simulink library "Blokk_Konyvtar"  (R2024b)
settings: Solver=VariableStepAuto  StartTime=0.0  StopTime=10.0  RelTol=1e-3
undefined symbols (not defined in the file or in its folder): __PRM__SERIALIZED__DATA__, Encoder, Sebessegmero
libraries: stm32f4xxblockslib x16, simulink x13, stm32blockslib x3, simulink_extras x2
settings Model: Creator=Asus  LastModifiedBy=Asus

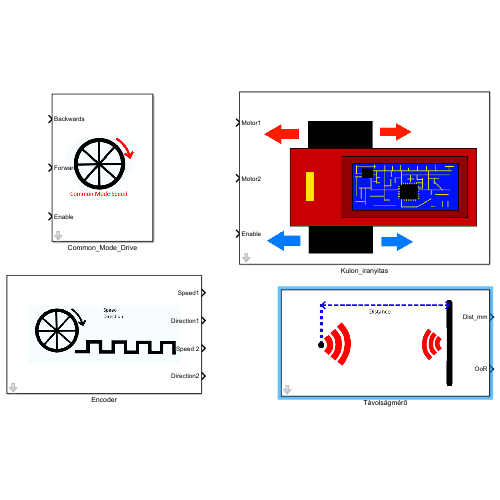
[thumbnail: Simulink's stored preview of the top-level diagram]
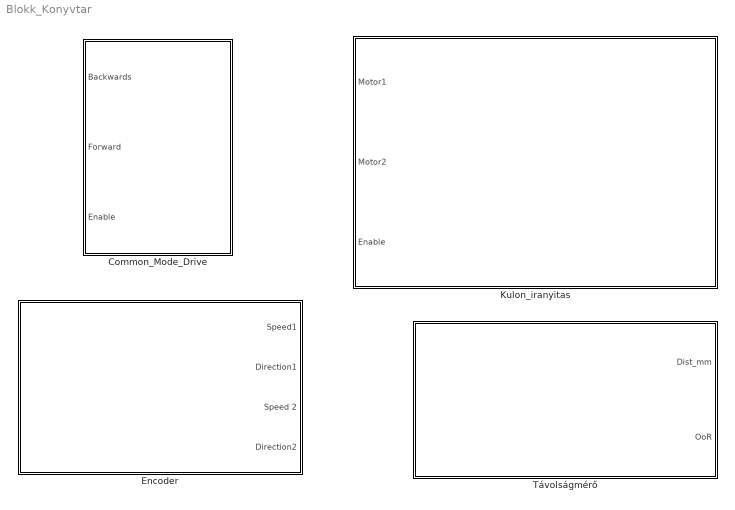
== system Blokk_Konyvtar ==
  Common_Mode_Drive : Subsystem
      mask DialogControl Control2 Prompt: This block applies common mode speed control for the wheels. The speed should be given in % value from 0-99.
      mask Display: image('Mask3_sebesseg.png', [20,20,20,20,100,100]);
  Encoder : Subsystem  BlockKeywords=__PRM__SERIALIZED__DATA__:Encoder,Sebessegmero  mask{TimClkFrq=25e6, CPR=1024, fwdvalue1=0, fwdvalue2=1, bckvalue1=1, bckvalue2=0, PrScaler=1}
      mask prompts: TimClkFrq "Timer Clock Frequency"; CPR "Counts Per Revolution"; fwdvalue1 "Forward Direction Value 1"; fwdvalue2 "Forward Direction Value 2"; bckvalue1 "Backward Direction Value 1"; bckvalue2 "Backward Direction Value 2"; PrScaler "Timer Prescaler (Shouldn't be Zero)"
      mask DialogControl DescTextVar Prompt: This block takes the encoder signal and converts it into speed and direction. The frequency of the timer channel and the counts per revolution is required to be filled with the correct values. The direction signals for each wheel is also customisable, thus the wheels may have a different base direction. The block uses Timer5 hardware interrupt on all 4 channels and reads PA0-3 GPIO ports. Modifying this requires looking under the mask.
      mask Display: image('Mask1.png', [30,10,30,10,100,100]);
  Kulon_iranyitas : Subsystem
      mask DialogControl Control2 Prompt: This block is meant for when you want to control the wheels independent of eachother. It can control the wheels with (-99;99) signals.
      mask Display: image('Maszk4_kulon_kerek.png', [25,25,5,0,100,100]);
  Távolságmérő : Subsystem  mask{TimClkFrq=1e8, PrScaler=50000, OoR_const=2000}
      mask prompts: TimClkFrq "Timer Frequency"; PrScaler "Timer Prescaler"; OoR_const "Out of Range distance [mm]"
      mask DialogControl DescTextVar Prompt: This block can be used to measure the distance of a ToF based sensor. The measured distance is in millimetres, and the user can configure an Out of Range signal.
      mask Display: image('Maszk2_tavmero.png', [30,10,40,10,100,100]);

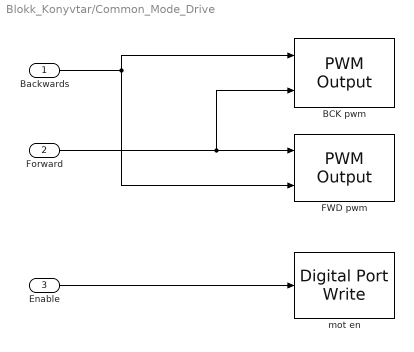
== system Blokk_Konyvtar/Common_Mode_Drive ==
  Backwards : Inport
  Forward : Inport  Port=2
  Enable : Inport  Port=3
  BCK pwm : stm32f4xxblockslib/PWM Output  TimerModule=TIM1  DutycycleUnits=Percentage  EnableChannel1=on  EnableChannel2=on  EnableChannel3=off  EnableChannel4=off  EnableCounterInput=off  EnableMainOutputInput=off  EnableFrequencyInput=off  SetRCAfterCE=off  OutputDirection=off  OutputMainOutputEnableStatus=off  SampleTime=0.1  EnableSimPort=off  EnableUpdateEvent=off  EnableCaptureCompare1Event=off  EnableCaptureCompare2Event=off  EnableCaptureCompare3Event=off  EnableCaptureCompare4Event=off  EnableTriggerEvent=off  EnableBreakEvent=off  ProcessorFamily=STM32F4  hoistedMaskSrc=ECSoC/ECSimCodegen/PWM Output
  "FWD pwm " : stm32f4xxblockslib/PWM Output  TimerModule=TIM3  DutycycleUnits=Percentage  EnableChannel1=off  EnableChannel2=off  EnableChannel3=on  EnableChannel4=on  EnableCounterInput=off  EnableMainOutputInput=off  EnableFrequencyInput=off  SetRCAfterCE=off  OutputDirection=off  OutputMainOutputEnableStatus=off  SampleTime=0.1  EnableSimPort=off  EnableUpdateEvent=off  EnableCaptureCompare1Event=off  EnableCaptureCompare2Event=off  EnableCaptureCompare3Event=off  EnableCaptureCompare4Event=off  EnableTriggerEvent=off  EnableBreakEvent=off  ProcessorFamily=STM32F4  hoistedMaskSrc=ECSoC/ECSimCodegen/PWM Output
  mot en : stm32f4xxblockslib/Digital Port Write  PortName=GPIOC  PinNumber=5  ReadOperation=off  IOAsArray=on  EnableSimPort=off  hoistedMaskSrc=ECSoC/ECSimCodegen/Digital Port Write
  wires:
  Forward/1 -> BCK pwm/2, "FWD pwm "/1
  Backwards/1 -> "FWD pwm "/2, BCK pwm/1
  Enable/1 -> mot en/1

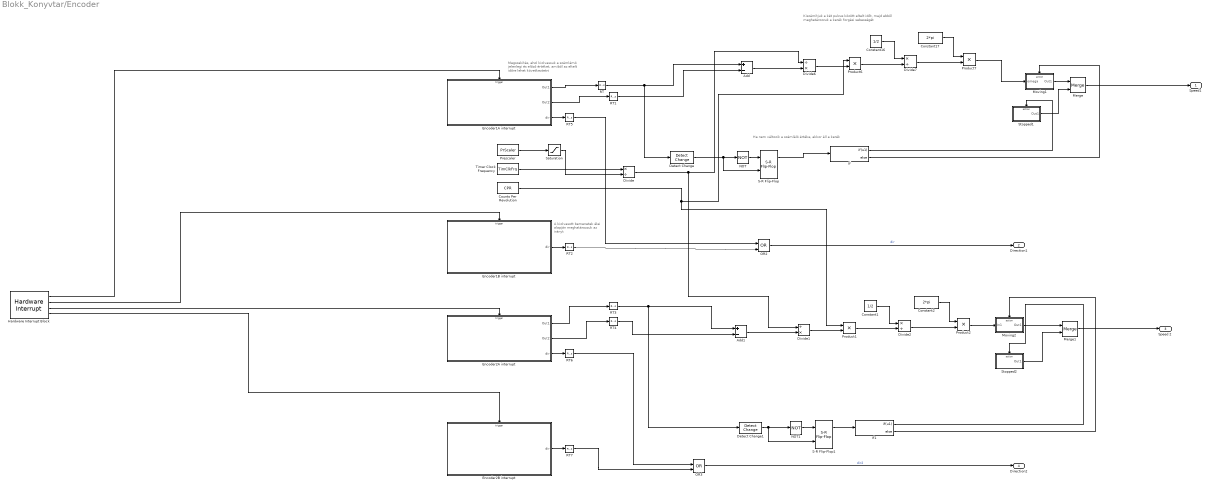
== system Blokk_Konyvtar/Encoder ==
  note: Kiszámítjuk a két pulzus között eltelt időt, majd ebből meghatározzuk a kerék forgási sebességét
  note: Ha nem változik a számláló értéke, akkor áll a kerék
  note: A kiolvasott bemenetek élei alapján meghatározzuk az irányt
  note: Megszakítás, ahol kiolvassuk a számlámó jelenlegi és előző értéket, amiből az eltelt időre lehet következtetni
  Add : Sum  Inputs=+-
  Add1 : Sum  Inputs=+-
  Constant1 : Constant  Value=1/2
  Constant16 : Constant  Value=1/2
  Constant17 : Constant  Value=2*pi
  Constant2 : Constant  Value=2*pi
  Counts Per Revolution : Constant  Value=CPR
  Detect Change : simulink/Logic and Bit Operations/Detect Change  vinit=0  OutDataTypeStr=boolean
  Detect Change1 : simulink/Logic and Bit Operations/Detect Change  vinit=0  OutDataTypeStr=boolean
  Divide : Product  Inputs=*/
  Divide1 : Product  Inputs=/*
  Divide2 : Product  Inputs=*/
  Divide6 : Product  Inputs=/*
  Divide7 : Product  Inputs=*/
  Encoder1A interrupt : Subsystem  TreatAsAtomicUnit=on
  Encoder1B interrupt : Subsystem  TreatAsAtomicUnit=on
  Encoder2A interrupt : Subsystem  TreatAsAtomicUnit=on
  Encoder2B interrupt : Subsystem  TreatAsAtomicUnit=on
  Hardware Interrupt Block : stm32f4xxblockslib/Hardware Interrupt  ISRGroup=Timer (TIM)  ISRName=TIM5_IRQHandler  ISRNumber=65  EventsList={ 'off', 'TIM5 Update', '1'; 'on', 'TIM5 CC1', '2'; 'on', 'TIM5 CC2', '3'; 'on', 'TIM5 CC3', '4'; 'on', 'TIM5 CC4', '5'; 'off', 'TIM5 Trigger', '6'; 'off', 'Custom event', '7' }  SelectedEvents={'TIM5 CC1','TIM5 CC2','TIM5 CC3','TIM5 CC4'}  TaskPriority=30  DisablePreemption=off  ClearInterruptFlagsAtEndOfEvent=on  InterruptDefinitionFile=$(TARGET_ROOT)/registry/interrupts/STM32F4xxBased_interrupts.xml  HardwareBoard=STM32F4xx Based  EnableSimPort=off
  If : If  IfExpression=u1
  If1 : If  IfExpression=u1
  Merge : Merge
  Merge1 : Merge
  Moving1 : Subsystem  TreatAsAtomicUnit=on
  Moving2 : Subsystem  TreatAsAtomicUnit=on
  NOT : Logic  Operator=NOT  IconShape=distinctive  AllPortsSameDT=off  OutDataTypeStr=boolean
  NOT1 : Logic  Operator=NOT  IconShape=distinctive  AllPortsSameDT=off  OutDataTypeStr=boolean
  OR2 : Logic  Operator=OR  IconShape=distinctive  AllPortsSameDT=off  OutDataTypeStr=boolean
  OR3 : Logic  Operator=OR  IconShape=distinctive  AllPortsSameDT=off  OutDataTypeStr=boolean
  Prescaler : Constant  Value=PrScaler
  Product{1..2,6..7} (4 alike) : Product
  RT{,1..7} (8 alike) : RateTransition  Deterministic=off  OutPortSampleTime=0.02
  S-R Flip-Flop : simulink_extras/Flip Flops/S-R Flip-Flop  initial_condition=0
  S-R Flip-Flop1 : simulink_extras/Flip Flops/S-R Flip-Flop  initial_condition=0
  Saturation : Saturate  UpperLimit=inf  LowerLimit=1
  Stopped1 : Subsystem  TreatAsAtomicUnit=on
  Stopped2 : Subsystem  TreatAsAtomicUnit=on
  Timer Clock Frequency : Constant  Value=TimClkFrq
  Speed1 : Outport
  Direction1 : Outport  Port=2
  Speed 2 : Outport  Port=3
  Direction2 : Outport  Port=4
  wires:
  S-R Flip-Flop1/1 -> If1/1
  Hardware Interrupt Block/4 -> Encoder2B interrupt/Trigger
  Encoder1A interrupt/2(Out2) -> RT1/1
  Product7/1 -> Moving1/1(omega)
  Stopped2/1(Out1) -> Merge1/2
  If/1 -> Stopped1/Action
  Moving1/1(Out1) -> Merge/1
  RT6/1 -> OR3/1
  If/2 -> Moving1/Action
  Hardware Interrupt Block/2 -> Encoder1B interrupt/Trigger
  Detect Change1/1 -> NOT1/1, S-R Flip-Flop1/2
  Hardware Interrupt Block/1 -> Encoder1A interrupt/Trigger
  Encoder2A interrupt/1(Out1) -> RT3/1
  If1/1 -> Stopped2/Action
  OR3/1 -> Direction2/1  "dir2"
  NOT/1 -> S-R Flip-Flop/1
  RT4/1 -> Add1/2
  Encoder2A interrupt/2(Out2) -> RT4/1
  Encoder1A interrupt/1(Out1) -> RT/1
  S-R Flip-Flop/1 -> If/1
  RT7/1 -> OR3/2
  Moving2/1(Out1) -> Merge1/1
  Hardware Interrupt Block/3 -> Encoder2A interrupt/Trigger
  If1/2 -> Moving2/Action
  RT/1 -> Add/1, Detect Change/1
  Stopped1/1(Out1) -> Merge/2
  RT3/1 -> Add1/1, Detect Change1/1
  RT5/1 -> OR2/1
  RT2/1 -> OR2/2
  NOT1/1 -> S-R Flip-Flop1/1
  Merge1/1 -> Speed 2/1
  Detect Change/1 -> NOT/1, S-R Flip-Flop/2
  Merge/1 -> Speed1/1
  RT1/1 -> Add/2
  Product2/1 -> Moving2/1(In1)
  OR2/1 -> Direction1/1  "dir"
  Encoder1B interrupt/1(dir) -> RT2/1
  Encoder1A interrupt/3(dir) -> RT5/1
  Encoder2A interrupt/3(dir) -> RT6/1
  Encoder2B interrupt/1(dir) -> RT7/1
  Timer Clock Frequency/1 -> Divide/1
  Prescaler/1 -> Saturation/1
  Divide/1 -> Divide1/1, Divide6/1
  Counts Per Revolution/1 -> Product1/1, Product6/1
  Product6/1 -> Divide7/2
  Divide7/1 -> Product7/2
  Divide6/1 -> Product6/2
  Add/1 -> Divide6/2
  Constant17/1 -> Product7/1
  Constant16/1 -> Divide7/1
  Saturation/1 -> Divide/2
  Divide1/1 -> Product1/2
  Add1/1 -> Divide1/2
  Constant1/1 -> Divide2/1
  Product1/1 -> Divide2/2
  Divide2/1 -> Product2/2
  Constant2/1 -> Product2/1

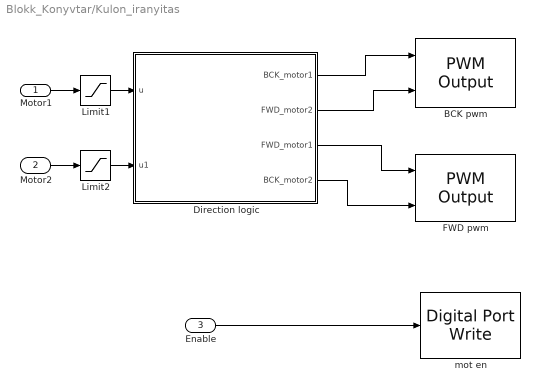
== system Blokk_Konyvtar/Kulon_iranyitas ==
  Motor1 : Inport
  Motor2 : Inport  Port=2
  Enable : Inport  Port=3
  BCK pwm : stm32f4xxblockslib/PWM Output  TimerModule=TIM1  DutycycleUnits=Percentage  EnableChannel1=on  EnableChannel2=on  EnableChannel3=off  EnableChannel4=off  EnableCounterInput=off  EnableMainOutputInput=off  EnableFrequencyInput=off  SetRCAfterCE=off  OutputDirection=off  OutputMainOutputEnableStatus=off  SampleTime=0.1  EnableSimPort=off  EnableUpdateEvent=off  EnableCaptureCompare1Event=off  EnableCaptureCompare2Event=off  EnableCaptureCompare3Event=off  EnableCaptureCompare4Event=off  EnableTriggerEvent=off  EnableBreakEvent=off  ProcessorFamily=STM32F4  hoistedMaskSrc=ECSoC/ECSimCodegen/PWM Output
  Direction logic : Subsystem
  "FWD pwm " : stm32f4xxblockslib/PWM Output  TimerModule=TIM3  DutycycleUnits=Percentage  EnableChannel1=off  EnableChannel2=off  EnableChannel3=on  EnableChannel4=on  EnableCounterInput=off  EnableMainOutputInput=off  EnableFrequencyInput=off  SetRCAfterCE=off  OutputDirection=off  OutputMainOutputEnableStatus=off  SampleTime=0.1  EnableSimPort=off  EnableUpdateEvent=off  EnableCaptureCompare1Event=off  EnableCaptureCompare2Event=off  EnableCaptureCompare3Event=off  EnableCaptureCompare4Event=off  EnableTriggerEvent=off  EnableBreakEvent=off  ProcessorFamily=STM32F4  hoistedMaskSrc=ECSoC/ECSimCodegen/PWM Output
  Limit1 : Saturate  UpperLimit=99  LowerLimit=-99
  Limit2 : Saturate  UpperLimit=99  LowerLimit=-99
  mot en : stm32f4xxblockslib/Digital Port Write  PortName=GPIOC  PinNumber=5  ReadOperation=off  IOAsArray=on  EnableSimPort=off  hoistedMaskSrc=ECSoC/ECSimCodegen/Digital Port Write
  wires:
  Enable/1 -> mot en/1
  Motor1/1 -> Limit1/1
  Motor2/1 -> Limit2/1
  Direction logic/1(BCK_motor1) -> BCK pwm/1
  Direction logic/2(FWD_motor2) -> BCK pwm/2
  Direction logic/3(FWD_motor1) -> "FWD pwm "/1
  Direction logic/4(BCK_motor2) -> "FWD pwm "/2
  Limit1/1 -> Direction logic/1(u)
  Limit2/1 -> Direction logic/2(u1)

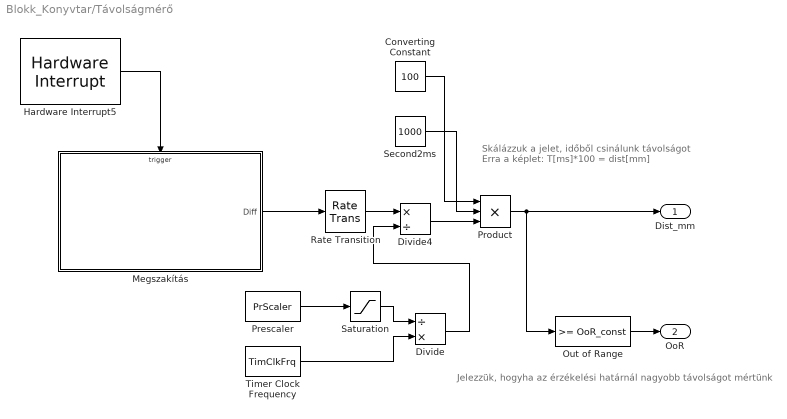
== system Blokk_Konyvtar/Távolságmérő ==
  note: Jelezzük, hogyha az érzékelési határnál nagyobb távolságot mértünk
  note: Skálázzuk a jelet, időből csinálunk távolságot
      | Erra a képlet: T[ms]*100 = dist[mm]
  Converting Constant : Constant  Value=100
  Divide : Product  Inputs=/*
  Divide4 : Product  Inputs=*/
  Hardware Interrupt5 : stm32f4xxblockslib/Hardware Interrupt  ISRGroup=Timer (TIM)  ISRName=TIM4_IRQHandler  ISRNumber=45  EventsList={ 'off', 'TIM4 Update', '1'; 'off', 'TIM4 CC1', '2'; 'on', 'TIM4 CC2', '3'; 'off', 'TIM4 CC3', '4'; 'off', 'TIM4 CC4', '5'; 'off', 'TIM4 Trigger', '6'; 'off', 'Custom event', '7' }  SelectedEvents={'TIM4 CC2'}  TaskPriority=30  DisablePreemption=off  ClearInterruptFlagsAtEndOfEvent=off  InterruptDefinitionFile=$(TARGET_ROOT)/registry/interrupts/STM32F4xxBased_interrupts.xml  HardwareBoard=STM32F4xx Based  EnableSimPort=off
  Megszakítás : Subsystem  TreatAsAtomicUnit=on
  Out of Range : simulink/Logic and Bit Operations/Compare To Constant  relop=>=  const=OoR_const  OutDataTypeStr=boolean
  Prescaler : Constant  Value=PrScaler
  Product : Product  Inputs=3
  Rate Transition : RateTransition  Deterministic=off  OutPortSampleTime=0.0001
  Saturation : Saturate  UpperLimit=inf  LowerLimit=1
  Second2ms : Constant  Value=1000
  Timer Clock Frequency : Constant  Value=TimClkFrq
  Dist_mm : Outport
  OoR : Outport  Port=2
  wires:
  Hardware Interrupt5/1 -> Megszakítás/Trigger
  Rate Transition/1 -> Divide4/1
  Out of Range/1 -> OoR/1
  Second2ms/1 -> Product/2
  Divide4/1 -> Product/3
  Prescaler/1 -> Saturation/1
  Divide/1 -> Divide4/2
  Saturation/1 -> Divide/1
  Converting Constant/1 -> Product/1
  Timer Clock Frequency/1 -> Divide/2
  Product/1 -> Out of Range/1, Dist_mm/1
  Megszakítás/1(Diff) -> Rate Transition/1

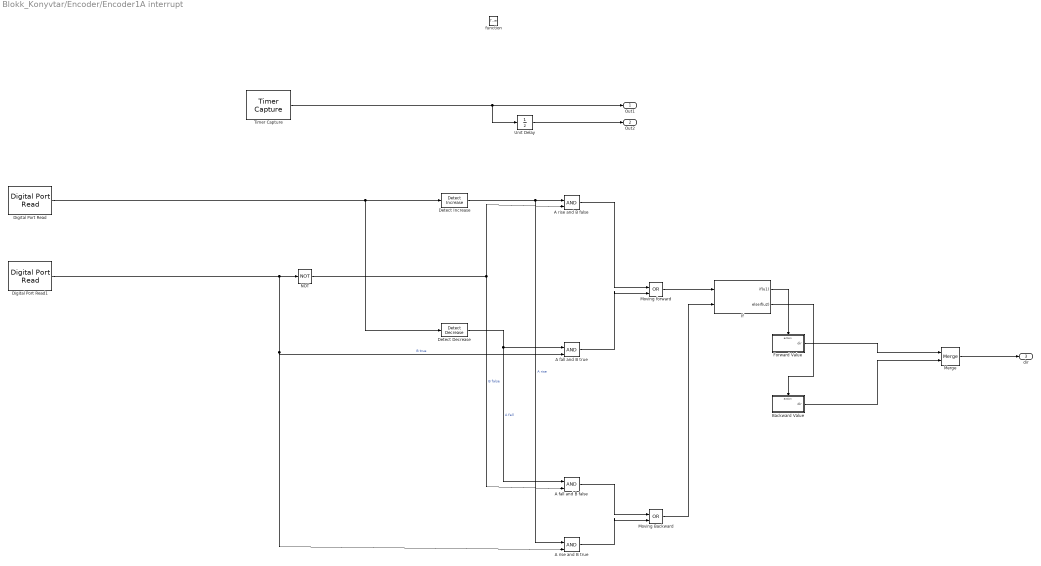
== system Blokk_Konyvtar/Encoder/Encoder1A interrupt ==
  function : TriggerPort  TriggerType=function-call  VariantControl=(inherit)
  A fall and B false : Logic  IconShape=distinctive  AllPortsSameDT=off  OutDataTypeStr=boolean
  A fall and B true : Logic  IconShape=distinctive  AllPortsSameDT=off  OutDataTypeStr=boolean
  A rise and B false : Logic  IconShape=distinctive  AllPortsSameDT=off  OutDataTypeStr=boolean
  A rise and B true : Logic  IconShape=distinctive  AllPortsSameDT=off  OutDataTypeStr=boolean
  Backward Value : Subsystem  TreatAsAtomicUnit=on
  Detect Decrease : simulink/Logic and Bit Operations/Detect Decrease  vinit=0.0  OutDataTypeStr=boolean
  Detect Increase : simulink/Logic and Bit Operations/Detect Increase  vinit=0.0  OutDataTypeStr=boolean
  Digital Port Read : stm32f4xxblockslib/Digital Port Read  PortName=GPIOA  PinNumber=[0]  ReadOperation=on  IOAsArray=on  SampleTime=-1  EnableSimPort=off  hoistedMaskSrc=ECSoC/ECSimCodegen/Digital Port Read
  Digital Port Read1 : stm32f4xxblockslib/Digital Port Read  PortName=GPIOA  PinNumber=[1]  ReadOperation=on  IOAsArray=on  SampleTime=-1  EnableSimPort=off  hoistedMaskSrc=ECSoC/ECSimCodegen/Digital Port Read
  Forward Value : Subsystem  TreatAsAtomicUnit=on
  If : If  NumInputs=2  IfExpression=u1  ElseIfExpressions=u2  ShowElse=off
  Merge : Merge
  Moving Backward : Logic  Operator=OR  IconShape=distinctive  AllPortsSameDT=off  OutDataTypeStr=boolean
  Moving forward : Logic  Operator=OR  IconShape=distinctive  AllPortsSameDT=off  OutDataTypeStr=boolean
  NOT : Logic  Operator=NOT  IconShape=distinctive  AllPortsSameDT=off  OutDataTypeStr=boolean
  Timer Capture : stm32blockslib/Timer Capture  TimerModule=TIM5  SelectedChannel=CH1  CaptureLength=1  OutputDataLength=off  OutputOverrunStatus=off  OutputDirection=off  SampleTime=-1
      settings: LibrarySourceBlock=stm32f4xxblockslib/Timer Capture
  Unit Delay : UnitDelay  SampleTime=-1  HasFrameUpgradeWarning=on
  Out1 : Outport
  Out2 : Outport  Port=2
  dir : Outport  Port=3
  wires:
  Timer Capture/1 -> Out1/1, Unit Delay/1
  Unit Delay/1 -> Out2/1
  If/1 -> Forward Value/Action
  If/2 -> Backward Value/Action
  A rise and B false/1 -> Moving forward/1
  A fall and B false/1 -> Moving Backward/1
  Moving forward/1 -> If/1
  A rise and B true/1 -> Moving Backward/2
  Forward Value/1(dir) -> Merge/1
  Digital Port Read/1 -> Detect Decrease/1, Detect Increase/1
  A fall and B true/1 -> Moving forward/2
  Digital Port Read1/1 -> A rise and B true/2, A fall and B true/2, NOT/1  "B true"
  Merge/1 -> dir/1
  Detect Increase/1 -> A rise and B true/1, A rise and B false/1  "A rise"
  NOT/1 -> A fall and B false/2, A rise and B false/2  "B false"
  Moving Backward/1 -> If/2
  Detect Decrease/1 -> A fall and B false/1, A fall and B true/1  "A fall"
  Backward Value/1(dir) -> Merge/2

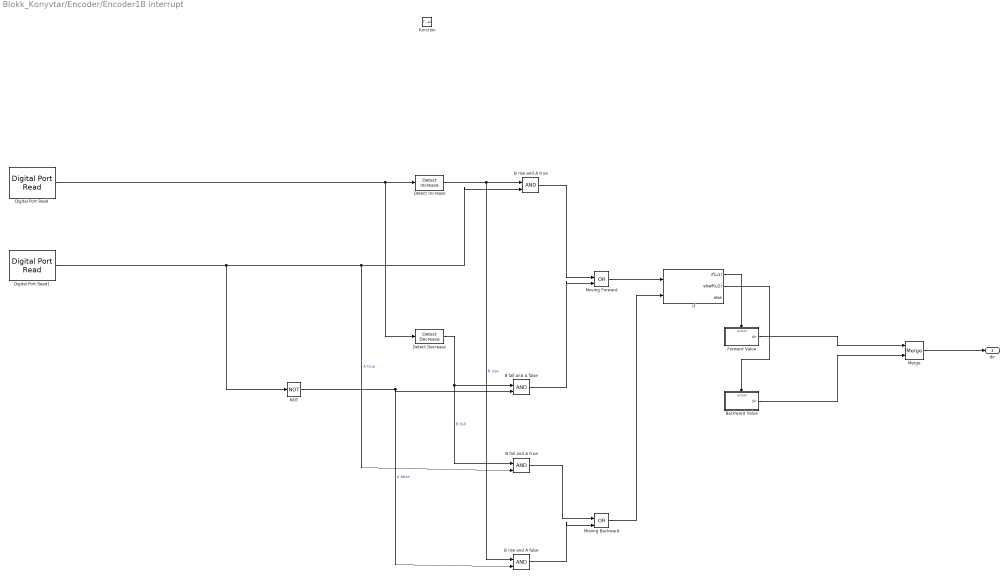
== system Blokk_Konyvtar/Encoder/Encoder1B interrupt ==
  function : TriggerPort  TriggerType=function-call  VariantControl=(inherit)
  B fall and A false : Logic  IconShape=distinctive  AllPortsSameDT=off  OutDataTypeStr=boolean
  B fall and A true : Logic  IconShape=distinctive  AllPortsSameDT=off  OutDataTypeStr=boolean
  B rise and A false : Logic  IconShape=distinctive  AllPortsSameDT=off  OutDataTypeStr=boolean
  B rise and A true : Logic  IconShape=distinctive  AllPortsSameDT=off  OutDataTypeStr=boolean
  Backward Value : Subsystem  TreatAsAtomicUnit=on
  Detect Decrease : simulink/Logic and Bit Operations/Detect Decrease  vinit=0.0  OutDataTypeStr=boolean
  Detect Increase : simulink/Logic and Bit Operations/Detect Increase  vinit=0.0  OutDataTypeStr=boolean
  Digital Port Read : stm32f4xxblockslib/Digital Port Read  PortName=GPIOA  PinNumber=[1]  ReadOperation=on  IOAsArray=on  SampleTime=-1  EnableSimPort=off  hoistedMaskSrc=ECSoC/ECSimCodegen/Digital Port Read
  Digital Port Read1 : stm32f4xxblockslib/Digital Port Read  PortName=GPIOA  PinNumber=[0]  ReadOperation=on  IOAsArray=on  SampleTime=-1  EnableSimPort=off  hoistedMaskSrc=ECSoC/ECSimCodegen/Digital Port Read
  Forward Value : Subsystem  TreatAsAtomicUnit=on
  If : If  NumInputs=2  IfExpression=u1  ElseIfExpressions=u2
  Merge : Merge
  Moving Backward : Logic  Operator=OR  IconShape=distinctive  AllPortsSameDT=off  OutDataTypeStr=boolean
  Moving Forward : Logic  Operator=OR  IconShape=distinctive  AllPortsSameDT=off  OutDataTypeStr=boolean
  NOT : Logic  Operator=NOT  IconShape=distinctive  AllPortsSameDT=off  OutDataTypeStr=boolean
  dir : Outport
  wires:
  Digital Port Read1/1 -> NOT/1, B rise and A true/2, B fall and A true/2  "A true"
  Moving Forward/1 -> If/1
  Backward Value/1(dir) -> Merge/2
  B fall and A false/1 -> Moving Forward/2
  B rise and A true/1 -> Moving Forward/1
  Digital Port Read/1 -> Detect Decrease/1, Detect Increase/1
  Detect Decrease/1 -> B fall and A true/1, B fall and A false/1  "B fall"
  Forward Value/1(dir) -> Merge/1
  Moving Backward/1 -> If/2
  If/2 -> Backward Value/Action
  B fall and A true/1 -> Moving Backward/1
  If/1 -> Forward Value/Action
  Merge/1 -> dir/1
  B rise and A false/1 -> Moving Backward/2
  NOT/1 -> B rise and A false/2, B fall and A false/2  "A false"
  Detect Increase/1 -> B rise and A false/1, B rise and A true/1  "B rise"

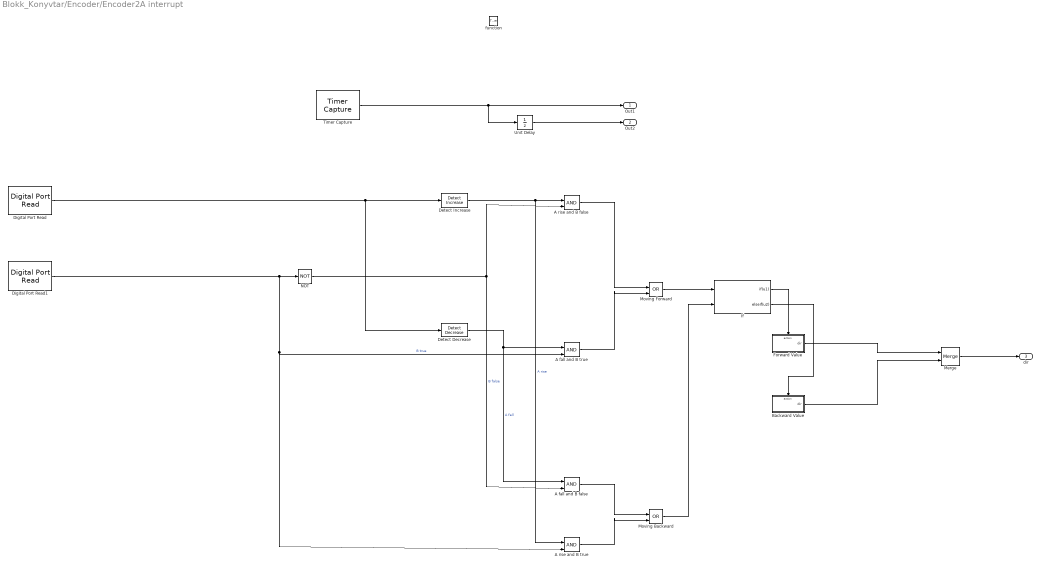
== system Blokk_Konyvtar/Encoder/Encoder2A interrupt ==
  function : TriggerPort  TriggerType=function-call  VariantControl=(inherit)
  A fall and B false : Logic  IconShape=distinctive  AllPortsSameDT=off  OutDataTypeStr=boolean
  A fall and B true : Logic  IconShape=distinctive  AllPortsSameDT=off  OutDataTypeStr=boolean
  A rise and B false : Logic  IconShape=distinctive  AllPortsSameDT=off  OutDataTypeStr=boolean
  A rise and B true : Logic  IconShape=distinctive  AllPortsSameDT=off  OutDataTypeStr=boolean
  Backward Value : Subsystem  TreatAsAtomicUnit=on
  Detect Decrease : simulink/Logic and Bit Operations/Detect Decrease  vinit=0.0  OutDataTypeStr=boolean
  Detect Increase : simulink/Logic and Bit Operations/Detect Increase  vinit=0.0  OutDataTypeStr=boolean
  Digital Port Read : stm32f4xxblockslib/Digital Port Read  PortName=GPIOA  PinNumber=[2]  ReadOperation=on  IOAsArray=on  SampleTime=-1  EnableSimPort=off  hoistedMaskSrc=ECSoC/ECSimCodegen/Digital Port Read
  Digital Port Read1 : stm32f4xxblockslib/Digital Port Read  PortName=GPIOA  PinNumber=[3]  ReadOperation=on  IOAsArray=on  SampleTime=-1  EnableSimPort=off  hoistedMaskSrc=ECSoC/ECSimCodegen/Digital Port Read
  Forward Value : Subsystem  TreatAsAtomicUnit=on
  If : If  NumInputs=2  IfExpression=u1  ElseIfExpressions=u2  ShowElse=off
  Merge : Merge
  Moving Backward : Logic  Operator=OR  IconShape=distinctive  AllPortsSameDT=off  OutDataTypeStr=boolean
  Moving Forward : Logic  Operator=OR  IconShape=distinctive  AllPortsSameDT=off  OutDataTypeStr=boolean
  NOT : Logic  Operator=NOT  IconShape=distinctive  AllPortsSameDT=off  OutDataTypeStr=boolean
  Timer Capture : stm32blockslib/Timer Capture  TimerModule=TIM5  SelectedChannel=CH3  CaptureLength=1  OutputDataLength=off  OutputOverrunStatus=off  OutputDirection=off  SampleTime=-1
      settings: LibrarySourceBlock=stm32f4xxblockslib/Timer Capture
  Unit Delay : UnitDelay  SampleTime=-1  HasFrameUpgradeWarning=on
  Out1 : Outport
  Out2 : Outport  Port=2
  dir : Outport  Port=3
  wires:
  Unit Delay/1 -> Out2/1
  If/1 -> Forward Value/Action
  If/2 -> Backward Value/Action
  A rise and B false/1 -> Moving Forward/1
  A fall and B false/1 -> Moving Backward/1
  Moving Forward/1 -> If/1
  A rise and B true/1 -> Moving Backward/2
  Forward Value/1(dir) -> Merge/1
  A fall and B true/1 -> Moving Forward/2
  Digital Port Read1/1 -> A rise and B true/2, A fall and B true/2, NOT/1  "B true"
  Merge/1 -> dir/1
  Detect Increase/1 -> A rise and B true/1, A rise and B false/1  "A rise"
  NOT/1 -> A fall and B false/2, A rise and B false/2  "B false"
  Moving Backward/1 -> If/2
  Detect Decrease/1 -> A fall and B false/1, A fall and B true/1  "A fall"
  Backward Value/1(dir) -> Merge/2
  Digital Port Read/1 -> Detect Increase/1, Detect Decrease/1
  Timer Capture/1 -> Unit Delay/1, Out1/1

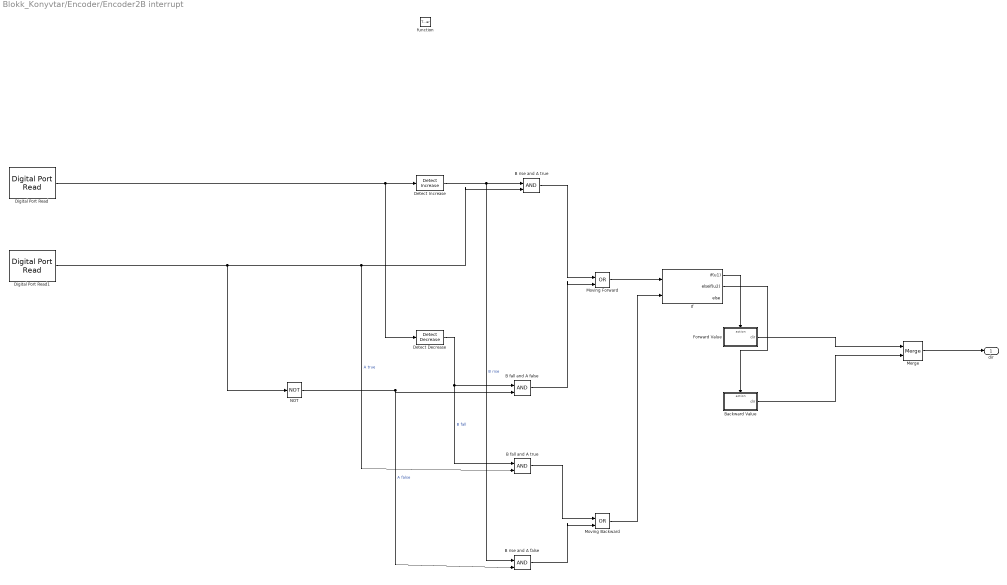
== system Blokk_Konyvtar/Encoder/Encoder2B interrupt ==
  function : TriggerPort  TriggerType=function-call  VariantControl=(inherit)
  B fall and A false : Logic  IconShape=distinctive  AllPortsSameDT=off  OutDataTypeStr=boolean
  B fall and A true : Logic  IconShape=distinctive  AllPortsSameDT=off  OutDataTypeStr=boolean
  B rise and A false : Logic  IconShape=distinctive  AllPortsSameDT=off  OutDataTypeStr=boolean
  B rise and A true : Logic  IconShape=distinctive  AllPortsSameDT=off  OutDataTypeStr=boolean
  Backward Value : Subsystem  TreatAsAtomicUnit=on
  Detect Decrease : simulink/Logic and Bit Operations/Detect Decrease  vinit=0.0  OutDataTypeStr=boolean
  Detect Increase : simulink/Logic and Bit Operations/Detect Increase  vinit=0.0  OutDataTypeStr=boolean
  Digital Port Read : stm32f4xxblockslib/Digital Port Read  PortName=GPIOA  PinNumber=[3]  ReadOperation=on  IOAsArray=on  SampleTime=-1  EnableSimPort=off  hoistedMaskSrc=ECSoC/ECSimCodegen/Digital Port Read
  Digital Port Read1 : stm32f4xxblockslib/Digital Port Read  PortName=GPIOA  PinNumber=[2]  ReadOperation=on  IOAsArray=on  SampleTime=-1  EnableSimPort=off  hoistedMaskSrc=ECSoC/ECSimCodegen/Digital Port Read
  Forward Value : Subsystem  TreatAsAtomicUnit=on
  If : If  NumInputs=2  IfExpression=u1  ElseIfExpressions=u2
  Merge : Merge
  Moving Backward : Logic  Operator=OR  IconShape=distinctive  AllPortsSameDT=off  OutDataTypeStr=boolean
  Moving Forward : Logic  Operator=OR  IconShape=distinctive  AllPortsSameDT=off  OutDataTypeStr=boolean
  NOT : Logic  Operator=NOT  IconShape=distinctive  AllPortsSameDT=off  OutDataTypeStr=boolean
  dir : Outport
  wires:
  Backward Value/1(dir) -> Merge/2
  Forward Value/1(dir) -> Merge/1
  If/2 -> Backward Value/Action
  If/1 -> Forward Value/Action
  Merge/1 -> dir/1
  Digital Port Read1/1 -> NOT/1, B rise and A true/2, B fall and A true/2  "A true"
  B rise and A false/1 -> Moving Backward/2
  Detect Decrease/1 -> B fall and A true/1, B fall and A false/1  "B fall"
  B fall and A true/1 -> Moving Backward/1
  Moving Forward/1 -> If/1
  NOT/1 -> B rise and A false/2, B fall and A false/2  "A false"
  Moving Backward/1 -> If/2
  B rise and A true/1 -> Moving Forward/1
  B fall and A false/1 -> Moving Forward/2
  Digital Port Read/1 -> Detect Decrease/1, Detect Increase/1
  Detect Increase/1 -> B rise and A false/1, B rise and A true/1  "B rise"

== system Blokk_Konyvtar/Encoder/Moving1 ==
  omega : Inport
  Action Port : ActionPort
  Out1 : Outport
  wires:
  omega/1 -> Out1/1

== system Blokk_Konyvtar/Encoder/Moving2 ==
  In1 : Inport
  Action Port : ActionPort
  Out1 : Outport
  wires:
  In1/1 -> Out1/1

== system Blokk_Konyvtar/Encoder/Stopped1 ==
  Action Port : ActionPort
  Constant : Constant  Value=0
  Out1 : Outport
  wires:
  Constant/1 -> Out1/1

== system Blokk_Konyvtar/Encoder/Stopped2 ==
  Action Port : ActionPort
  Constant : Constant  Value=0
  Out1 : Outport
  wires:
  Constant/1 -> Out1/1

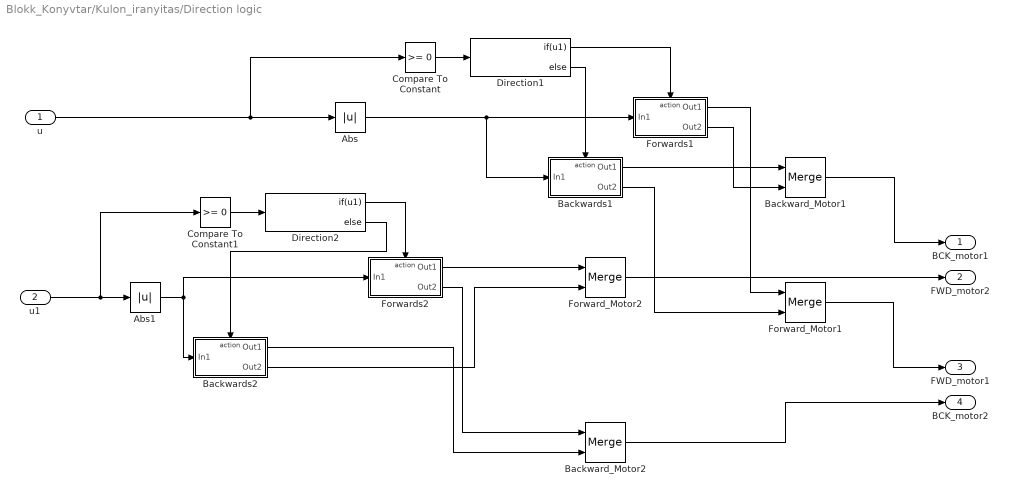
== system Blokk_Konyvtar/Kulon_iranyitas/Direction logic ==
  u : Inport
  u1 : Inport  Port=2
  Abs : Abs  SaturateOnIntegerOverflow=off
  Abs1 : Abs  SaturateOnIntegerOverflow=off
  Backward_Motor1 : Merge
  Backward_Motor2 : Merge
  Backwards1 : Subsystem  TreatAsAtomicUnit=on
  Backwards2 : Subsystem  TreatAsAtomicUnit=on
  Compare To Constant : simulink/Logic and Bit Operations/Compare To Constant  relop=>=  const=0  OutDataTypeStr=boolean
  Compare To Constant1 : simulink/Logic and Bit Operations/Compare To Constant  relop=>=  const=0  OutDataTypeStr=boolean
  Direction1 : If  IfExpression=u1
  Direction2 : If  IfExpression=u1
  Forward_Motor1 : Merge
  Forward_Motor2 : Merge
  Forwards1 : Subsystem  TreatAsAtomicUnit=on
  Forwards2 : Subsystem  TreatAsAtomicUnit=on
  BCK_motor1 : Outport
  FWD_motor2 : Outport  Port=2
  FWD_motor1 : Outport  Port=3
  BCK_motor2 : Outport  Port=4
  wires:
  Forward_Motor2/1 -> FWD_motor2/1
  Forwards1/1(Out1) -> Forward_Motor1/1
  Backwards1/1(Out1) -> Backward_Motor1/1
  Backwards2/2(Out2) -> Forward_Motor2/2
  Compare To Constant/1 -> Direction1/1
  Direction1/2 -> Backwards1/Action
  Direction1/1 -> Forwards1/Action
  Backwards2/1(Out1) -> Backward_Motor2/2
  Abs1/1 -> Forwards2/1(In1), Backwards2/1(In1)
  Abs/1 -> Backwards1/1(In1), Forwards1/1(In1)
  Forwards1/2(Out2) -> Backward_Motor1/2
  u/1 -> Compare To Constant/1, Abs/1
  Backward_Motor2/1 -> BCK_motor2/1
  Direction2/1 -> Forwards2/Action
  Compare To Constant1/1 -> Direction2/1
  u1/1 -> Compare To Constant1/1, Abs1/1
  Backward_Motor1/1 -> BCK_motor1/1
  Direction2/2 -> Backwards2/Action
  Backwards1/2(Out2) -> Forward_Motor1/2
  Forwards2/1(Out1) -> Forward_Motor2/1
  Forwards2/2(Out2) -> Backward_Motor2/1
  Forward_Motor1/1 -> FWD_motor1/1

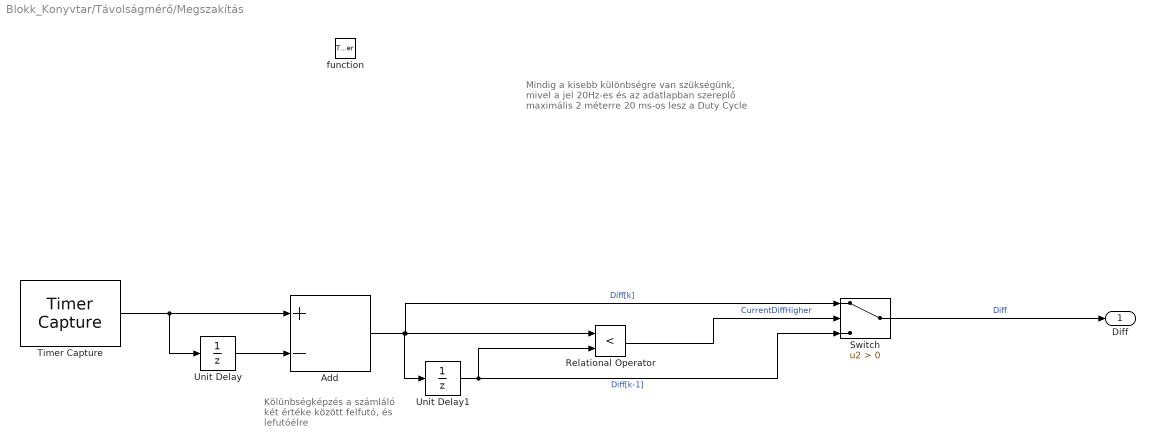
== system Blokk_Konyvtar/Távolságmérő/Megszakítás ==
  note: Mindig a kisebb különbségre van szükségünk, mivel a jel 20Hz-es és az adatlapban szereplő maximális 2 méterre 20 ms-os lesz a Duty Cycle
  note: Kölünbségképzés a számláló két értéke között felfutó, és lefutóélre
  function : TriggerPort  TriggerType=function-call  VariantControl=(inherit)
  Add : Sum  Inputs=+-
  Relational Operator : RelationalOperator  Operator=<  OutDataTypeStr=boolean  RndMeth=Simplest  InputSameDT=off
  Switch : Switch  Criteria=u2 > Threshold  SaturateOnIntegerOverflow=off  InputSameDT=off
  Timer Capture : stm32blockslib/Timer Capture  TimerModule=TIM4  SelectedChannel=CH2  CaptureLength=1  OutputDataLength=off  OutputOverrunStatus=off  OutputDirection=off  SampleTime=-1
  Unit Delay : UnitDelay  SampleTime=-1  HasFrameUpgradeWarning=on
  Unit Delay1 : UnitDelay  SampleTime=-1  HasFrameUpgradeWarning=on
  Diff : Outport
  wires:
  Add/1 -> Switch/1, Relational Operator/1, Unit Delay1/1  "Diff[k]"
  Timer Capture/1 -> Unit Delay/1, Add/1
  Unit Delay1/1 -> Switch/3, Relational Operator/2  "Diff[k-1]"
  Relational Operator/1 -> Switch/2  "CurrentDiffHigher"
  Switch/1 -> Diff/1  "Diff"
  Unit Delay/1 -> Add/2

== system Blokk_Konyvtar/Encoder/Encoder1A interrupt/Backward Value ==
  Action Port : ActionPort
  Constant : Constant  Value=bckvalue1
  dir : Outport
  wires:
  Constant/1 -> dir/1

== system Blokk_Konyvtar/Encoder/Encoder1A interrupt/Forward Value ==
  Action Port : ActionPort
  Constant : Constant  Value=fwdvalue1
  dir : Outport
  wires:
  Constant/1 -> dir/1

== system Blokk_Konyvtar/Encoder/Encoder1B interrupt/Backward Value ==
  Action Port : ActionPort
  Constant : Constant  Value=bckvalue1
  dir : Outport
  wires:
  Constant/1 -> dir/1

== system Blokk_Konyvtar/Encoder/Encoder1B interrupt/Forward Value ==
  Action Port : ActionPort
  Constant : Constant  Value=fwdvalue1
  dir : Outport
  wires:
  Constant/1 -> dir/1

== system Blokk_Konyvtar/Encoder/Encoder2A interrupt/Backward Value ==
  Action Port : ActionPort
  Constant : Constant  Value=bckvalue2
  dir : Outport
  wires:
  Constant/1 -> dir/1

== system Blokk_Konyvtar/Encoder/Encoder2A interrupt/Forward Value ==
  Action Port : ActionPort
  Constant : Constant  Value=fwdvalue2
  dir : Outport
  wires:
  Constant/1 -> dir/1

== system Blokk_Konyvtar/Encoder/Encoder2B interrupt/Backward Value ==
  Action Port : ActionPort
  Constant : Constant  Value=bckvalue2
  dir : Outport
  wires:
  Constant/1 -> dir/1

== system Blokk_Konyvtar/Encoder/Encoder2B interrupt/Forward Value ==
  Action Port : ActionPort
  Constant : Constant  Value=fwdvalue2
  dir : Outport
  wires:
  Constant/1 -> dir/1

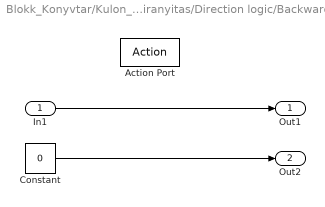
== system Blokk_Konyvtar/Kulon_iranyitas/Direction logic/Backwards1 ==
  In1 : Inport
  Action Port : ActionPort
  Constant : Constant  Value=0
  Out1 : Outport
  Out2 : Outport  Port=2
  wires:
  In1/1 -> Out1/1
  Constant/1 -> Out2/1

== system Blokk_Konyvtar/Kulon_iranyitas/Direction logic/Backwards2 ==
  In1 : Inport
  Action Port : ActionPort
  Constant : Constant  Value=0
  Out1 : Outport
  Out2 : Outport  Port=2
  wires:
  In1/1 -> Out1/1
  Constant/1 -> Out2/1

== system Blokk_Konyvtar/Kulon_iranyitas/Direction logic/Forwards1 ==
  In1 : Inport
  Action Port : ActionPort
  Constant : Constant  Value=0
  Out1 : Outport
  Out2 : Outport  Port=2
  wires:
  In1/1 -> Out1/1
  Constant/1 -> Out2/1

== system Blokk_Konyvtar/Kulon_iranyitas/Direction logic/Forwards2 ==
  In1 : Inport
  Action Port : ActionPort
  Constant : Constant  Value=0
  Out1 : Outport
  Out2 : Outport  Port=2
  wires:
  In1/1 -> Out1/1
  Constant/1 -> Out2/1
